simulink model "pendulum_sim2"  (Simulink 10.0)
settings: Solver=ode45  StartTime=0.0  StopTime=T_fin  MaxStep=T_step  RelTol=1e-3
values from neighbouring files (symbols this model uses):
  K = place(AAA, BBB, [-5 -4])    [main_inverted_pendulum.m]
  u_bar = [0]    [main_inverted_pendulum.m]
  x0 = [pi - epsi, 0]    [main_inverted_pendulum.m]
  x_bar = [pi, 0]    [main_inverted_pendulum.m]
undefined symbols (not defined in the file or in its folder): pendulum
settings Model: Creator=user  LastModifiedBy=user
settings DataIOCC: SaveFormat=Dataset  ReturnWorkspaceOutputs=on
settings OptimizationCC: LifeSpan=auto
settings DebuggingCC: UnderspecifiedInitializationDetection=Simplified  MergeDetectMultiDrivingBlocksExec=error  SFUnexpectedBacktrackingDiag=error  SFNoUnconditionalDefaultTransitionDiag=error  SFExecutionAtInitializationDiag=warning  ArithmeticOperatorsInVariantConditions=error
settings HardwareCC: ProdBitPerPointer=64  ProdBitPerSizeT=64  ProdBitPerPtrDiffT=64  ProdLargestAtomicFloat=Float  ProdIntDivRoundTo=Zero  ProdEndianess=LittleEndian  ProdWordSize=64  ProdHWDeviceType=Intel->x86-64 (Windows64)
settings ModelReferenceCC: PropagateSignalLabelsOutOfModel=on
settings SFSimCC: SimUseLocalCustomCode=on  CustomCodeUndefinedFunction=FilterOut
settings RTWCC: RTWUseLocalCustomCode=on
settings CodeAppCC: StateflowObjectComments=off
settings GRTTargetCC: TargetLangStandard=C99 (ISO)  CombineOutputUpdateFcns=on  GRTInterface=off
settings ConfigComp: CovMetricSettings=dwe  CovHtmlReporting=off  CovSaveCumulativeToWorkspaceVar=off  CovSaveSingleToWorkspaceVar=off

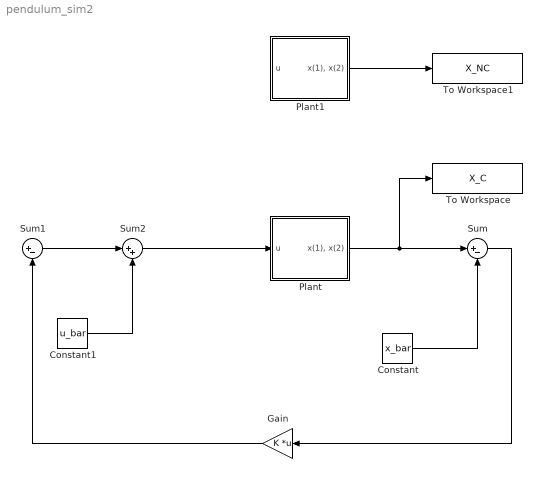
== system pendulum_sim2 ==
  Constant : Constant  Value=x_bar
  Constant1 : Constant  Value=u_bar
  Gain : Gain  Gain=K  Multiplication=Matrix(K*u)
  Plant : Subsystem
  Plant1 : Subsystem
  Sum : Sum  Inputs=|+-
  Sum1 : Sum  Inputs=|+-
  Sum2 : Sum  Inputs=|++
  To Workspace : ToWorkspace  VariableName=X_C  SampleTime=-1
  To Workspace1 : ToWorkspace  VariableName=X_NC  SampleTime=-1
  wires:
  Plant/1("x(1), x(2)") -> To Workspace/1, Sum/1
  Constant/1 -> Sum/2
  Sum/1 -> Gain/1
  Gain/1 -> Sum1/2
  Sum1/1 -> Sum2/1
  Constant1/1 -> Sum2/2
  Sum2/1 -> Plant/1(u)
  Plant1/1("x(1), x(2)") -> To Workspace1/1

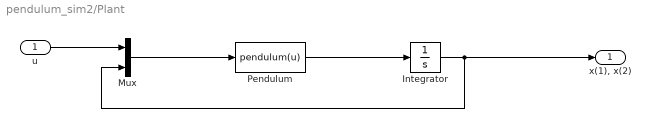
== system pendulum_sim2/Plant ==
  u : Inport
  Integrator : Integrator  InitialCondition=x0
  Mux : Mux  Inputs=2
  Pendulum : MATLABFcn  MATLABFcn=pendulum(u)
  "x(1), x(2)" : Outport
  wires:
  Mux/1 -> Pendulum/1
  Integrator/1 -> "x(1), x(2)"/1, Mux/2
  Pendulum/1 -> Integrator/1
  u/1 -> Mux/1

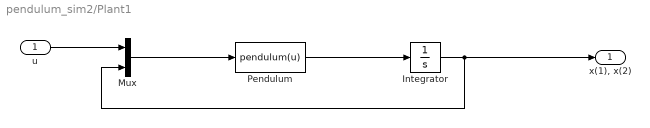
== system pendulum_sim2/Plant1 ==
  u : Inport
  Integrator : Integrator  InitialCondition=x0
  Mux : Mux  Inputs=2
  Pendulum : MATLABFcn  MATLABFcn=pendulum(u)
  "x(1), x(2)" : Outport
  wires:
  Mux/1 -> Pendulum/1
  Integrator/1 -> "x(1), x(2)"/1, Mux/2
  Pendulum/1 -> Integrator/1
  u/1 -> Mux/1
